simulink model "TVCVehicleModelAndSimulation_AreaVersion"  (R2024a)
settings: Solver=VariableStepAuto  StartTime=0.0  StopTime=20  RelTol=1e-3
values from neighbouring files (symbols this model uses):
  Gravity_Vector_Inertial = [0,0,Mass*9.81]    [ModelVariables.m]
  Thrust_Moment_Arm = 0.1    [ModelVariables.m]
  z_Reference = 30    [ModelVariables.m]
libraries: simulink_extras x2, shared6dof x1, slpidlib x1
settings Model: Creator=Joshua Caratao  LastModifiedBy=Joshua Caratao

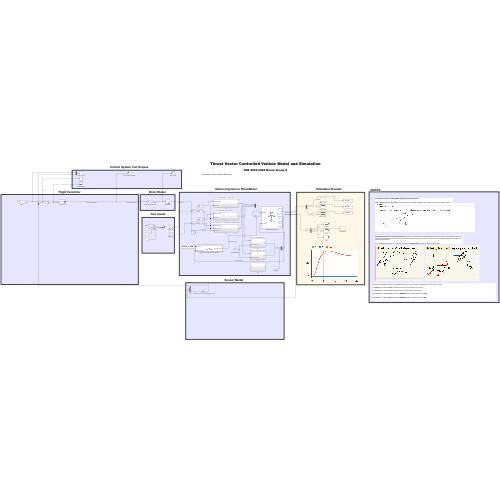
[thumbnail: Simulink's stored preview of the top-level diagram]
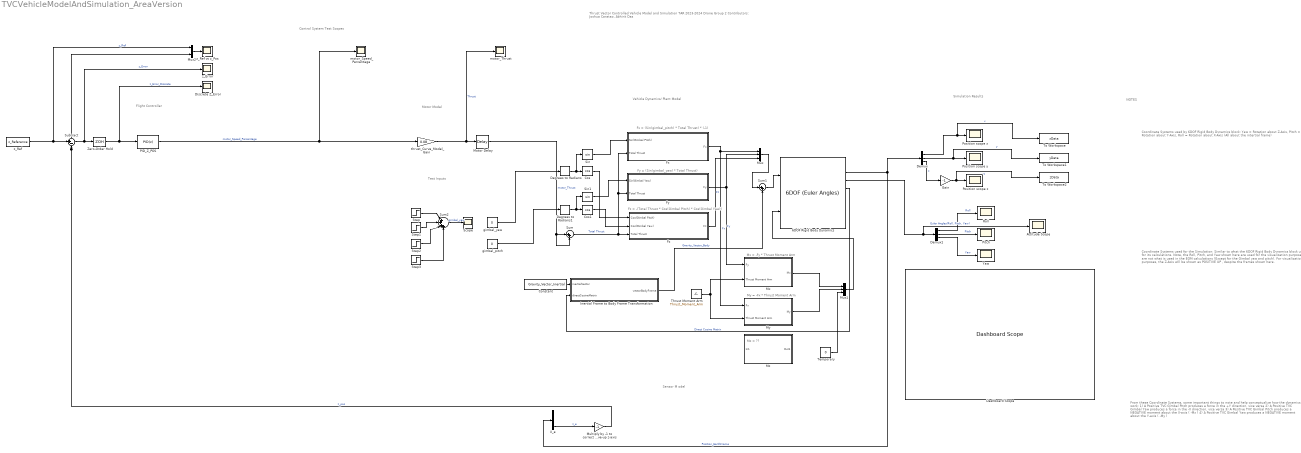
== system TVCVehicleModelAndSimulation_AreaVersion ==
  note: From these Coordinate Systems, some important things to note and help conceptualize how the dynamics work:
      |
      | 1) A Positive TVC Gimbal Pitch produces a force in the +Y direction, vice versa
      |
      | 2) A Positive TVC Gimbal Yaw produces a force in the -X direction, vice versa
      |
      | 3) A Positive TVC Gimbal Pitch produces a NEGATIVE moment about the X-axis ( -Mx )
      |
      | 4) A Positive TVC Gimbal Yaw produces a NEGATIVE moment about the Y-axis ( -My )
  note: NOTES
  note: Coordinate Systems used by 6DOF Rigid Body Dynamics block:
      |
      | Yaw = Rotation about Z-Axis, Pitch = Rotation about Y-Axis, Roll = Rotation about X-Axis (All about the intertial frame)
  note: Coordinate Systems used for the Simulation: Similar to what the 6DOF Rigid Body Dynamics block uses for its calculations. Note, the Roll, Pitch, and Yaw shown here are used for the visualization purposes and are not what is used in the EOM calculations (Except for the Gimbal yaw and pitch).
      |
      | For visualization purposes, the Z-Axis will be shown as POSITIVE UP , despite the frames shown here.
  note: Flight Controller
  note: Sensor M odel
  note: Vehicle Dynamics/ Plant Model
  note: Thrust Vector Controlled Vehicle Model and Simulation
      |
      | TAR 2023-2024 Drone Group 2
      |
      | Contributors: Joshua Caratao, Abhirit Das
  note: Fy = (Sin(gimbal_yaw) * Total Thrust)
  note: My = -Fx * Thrust Moment Arm
  note: Fx = (Sin(gimbal_pitch) * Total Thrust) * (-1)
  note: Mz = ??
  note: Fz = -(Total Thrust * Cos(Gimbal Pitch) * Cos(Gimbal Yaw))
  note: Mx = -Fy * Thrust Moment Arm
  note: Simulation Results
  note: Test Inputs
  note: Motor Model
  note: Control System Test Scopes
  "6DOF Rigid Body Dynamics " : shared6dof/6DOF (Euler Angles)  units=Metric (MKS)  mtype=Fixed  rep=Euler Angles  xme_0=Initial_Pos_Inertial_Axes  Vm_0=Initial_Vel_Body_Axes  eul_0=Initial_Euler_Orientation  pm_0=Initial_Body_Rotation_Rates  mass_0=Mass  mass_e=0.5  mass_f=2.0  inertia=Inertia_Tensor  inertia_e=eye(3)  inertia_f=2*eye(3)  k_quat=1.0  vre_flag=on  abi_flag=off  aMode=0  xme_statename=''  Vm_statename=''  eul_statename=''  quat_statename=''  pm_statename=''  mass_statename=''
  Attitude Scope : Scope
  Constant : Constant  Value=Gravity_Vector_Inertial
  Cos : Trigonometry  Operator=cos
  Cos1 : Trigonometry  Operator=cos
  Dashboard Scope : DashboardScope
  Degrees to Radians : simulink_extras/Transformations/Degrees to Radians
  Degrees to Radians1 : simulink_extras/Transformations/Degrees to Radians
  Demux : Demux  Outputs=3
  Demux1 : Demux  Outputs=3
  Discrete Z_Error : Scope
  Fx : Subsystem
  Fy : Subsystem
  Fz : Subsystem
  Gain : Gain  Gain=-1
  Inertial Frame to Body Frame Transformation : MATLAB Function  TreatAsAtomicUnit=on
  Motor Delay : TransportDelay  DelayTime=0.01
  Multiply by -1 to correct for a positive-up z-axis : Gain  Gain=-1
  Mux : Mux  Inputs=3
  Mux1 : Mux  Inputs=3
  Mux2 : Mux  Inputs=2
  Mx : Subsystem
  My : Subsystem
  Mz : Subsystem
  PID_Z_POS : slpidlib/PID Controller  Controller=PID  Form=Parallel  TimeDomain=Discrete-time  UseExternalTs=off  SampleTime=-1  IntegratorMethod=Forward Euler  FilterMethod=Forward Euler  ControllerParametersSource=internal  P=20  I=4  UseKiTs=off  D=40  UseExternalDerivativeSource=off  N=0  UseFilter=off  TunerSelectOption=Transfer Function Based (PID Tuner App)  InitialConditionSource=internal  InitialConditionForIntegrator=0  InitialConditionForFilter=0  DifferentiatorICPrevScaledInput=0  ExternalReset=none  TrackingMode=off  Kt=1  LimitOutput=on  SatLimitsSource=internal  UpperSaturationLimit=100  LowerSaturationLimit=0  LinearizeAsGain=off  AntiWindupMode=none  Kb=1  LimitIntegrator=off  UpperIntegratorSaturationLimit=2000  LowerIntegratorSaturationLimit=1000  POutMin=[]  POutMax=[]  IOutMin=[]  IOutMax=[]  DOutMin=[]  DOutMax=[]  NOutMin=[]  NOutMax=[]  SumOutMin=[]  SumOutMax=[]  SaturationOutMin=[]  SaturationOutMax=[]  PParamMin=[]  PParamMax=[]  IParamMin=[]  IParamMax=[]  DParamMin=[]  DParamMax=[]  NParamMin=[]  NParamMax=[]  KbParamMin=[]  KbParamMax=[]  KtParamMin=[]  KtParamMax=[]  KbOutMin=[]  KbOutMax=[]  KtOutMin=[]  KtOutMax=[]  IntegratorOutMin=[]  IntegratorOutMax=[]  FilterOutMin=[]  FilterOutMax=[]  SumI1OutMin=[]  SumI1OutMax=[]  SumI2OutMin=[]  SumI2OutMax=[]  SumI3OutMin=[]  SumI3OutMax=[]  SumI4OutMin=[]  SumI4OutMax=[]  SumDOutMin=[]  SumDOutMax=[]  DifferentiatorOutMin=[]  DifferentiatorOutMax=[]  FilterDiffOutCoefMin=[]  FilterDiffOutCoefMax=[]  ReciprocalOutMin=[]  ReciprocalOutMax=[]  SumDenOutMin=[]  SumDenOutMax=[]  SumNumOutMin=[]  SumNumOutMax=[]  DivideOutMin=[]  DivideOutMax=[]  UdiffTsProdOutMin=[]  UdiffTsProdOutMax=[]  NTsProdOutMin=[]  NTsProdOutMax=[]  UintegralTsProdOutMin=[]  UintegralTsProdOutMax=[]  UngainTsProdOutMin=[]  UngainTsProdOutMax=[]  ClampingZeroOutDataTypeStr=Inherit: Inherit via back propagation  ClampingZeroOutMin=[]  ClampingZeroOutMax=[]  FilterDenConstantOutDataTypeStr=Inherit: Inherit via back propagation  FilterDenConstantOutMin=[]  FilterDenConstantOutMax=[]  PCopyOutDataTypeStr=Inherit: Inherit via back propagation  PCopyOutMin=[]  PCopyOutMax=[]  NCopyOutDataTypeStr=Inherit: Inherit via back propagation  NCopyOutMin=[]  NCopyOutMax=[]  IntegratorContinuousStateAttributes=''  IntegratorStateMustResolveToSignalObject=off  IntegratorRTWStateStorageClass=Auto  FilterContinuousStateAttributes=''  FilterStateMustResolveToSignalObject=off  FilterRTWStateStorageClass=Auto  ParallelPVariant=InternalParameters  IdealPVariant=Disabled  IVariant=InternalParameters  DVariant=InternalParameters  IntegratorVariant=Discrete  SatVariant=Enabled  AWVariant=Passthrough  PCopyVariant=Disabled  TRVariant=Disabled  FdbkBlocksVariant=Forward  IdealPFdbkVariant=Disabled  SatFdbkVariant=Disabled  DerivativeFilterVariant=Differentiator  NVariant=Passthrough  NCopyVariant=Disabled_SignalSpec  FilterICVariant=InternalICsDifferentiator  IntegratorICVariant=InternalICs  ExternalResetVariant=Disabled  TRSumVariant=Passthrough  SumFdbkVariant=Disabled  SumVariant=Sum_PID  TsampFilterVariant=InternalTs  TsampNgainVariant=Passthrough  TsampIntegralVariant=Disabled_SignalSpec  ExternalSaturationOutDataTypeStr=Inherit: Same as second input  DerivativeSourceVariant=ErrorSignal
      settings: LibrarySourceBlock=simulink/Discrete/Discrete PID Controller
  Pitch : Scope
  Position scope x : Scope
  Position scope y : Scope
  Position scope z : Scope
  Roll : Scope
  Scope : Scope
  Sin : Trigonometry
  Sin1 : Trigonometry
  Step : Step  SampleTime=0
  Step1 : Step  Time=2  After=-1  SampleTime=0
  Step2 : Step  Time=3  After=-1.5  SampleTime=0
  Step3 : Step  Time=4  After=1.5  SampleTime=0
  Subtract : Sum  Inputs=|+-
  Sum : Sum  Inputs=|++
  Sum1 : Sum  Inputs=|++
  Sum2 : Sum  Inputs=|++++
  Temporary : Constant  Value=0
  "Thrust Moment Arm " : Constant  Value=Thrust_Moment_Arm
  To Workspace : ToWorkspace  VariableName=xData  SampleTime=-1
  To Workspace1 : ToWorkspace  VariableName=yData  SampleTime=-1
  To Workspace2 : ToWorkspace  VariableName=zData  SampleTime=-1
  X_e : Demux  Outputs=3
  Yaw : Scope
  Zero-Order Hold : ZeroOrderHold  SampleTime=0.01
  gimbal_pitch : Constant  Value=0
  gimbal_yaw : Constant  Value=0
  motor_Speed_Percentage : Scope
  motor_Thrust : Scope
  thrust_Curve_Model_Gain : Gain  Gain=0.08
  z_Error : Scope
  z_Ref : Constant  Value=z_Reference
  z_Ref vs z_Pos : Scope
  wires:
  "6DOF Rigid Body Dynamics "/3 -> Attitude Scope/1, Demux1/1  "Euler Angles(Roll, Pitch, Yaw)"
  "6DOF Rigid Body Dynamics "/2 -> X_e/1, Demux/1  "Position_EarthFrame"
  Demux/1 -> To Workspace/1, Position scope x/1  "x"
  Demux/2 -> To Workspace1/1, Position scope y/1  "y"
  Demux/3 -> Gain/1  "z"
  Temporary/1 -> Mux1/3
  "Thrust Moment Arm "/1 -> Mx/2(Thrust Moment Arm), My/2(Thrust Moment Arm)
  My/1(My) -> Mux1/2
  Sin1/1 -> Fy/1(Sin(Gimbal Yaw))
  Fz/1(Fz) -> Mux/3  "Fz"
  Cos1/1 -> Fz/2(Cos(Gimbal Yaw))
  Cos/1 -> Fz/1(Cos(Gimbal Pitch))
  Mx/1(Mx) -> Mux1/1
  Degrees to Radians1/1 -> Sin1/1, Cos1/1
  Sum2/1 -> Scope/1  "gimbal_yaw"
  Mux1/1 -> "6DOF Rigid Body Dynamics "/2
  Fy/1(Fy) -> Mux/2, Mx/1(Fy)  "Fy"
  gimbal_pitch/1 -> Degrees to Radians1/1
  Mux/1 -> Sum1/1
  Sum/1 -> Fz/3(Total Thrust), Fx/2(Total Thrust), Fy/2(Total Thrust)  "Total Thrust"
  Sin/1 -> Fx/1(Sin(Gimbal Pitch))
  Degrees to Radians/1 -> Sin/1, Cos/1
  Fx/1(Fx) -> Mux/1, My/1(Fx)  "Fx"
  thrust_Curve_Model_Gain/1 -> Motor Delay/1, motor_Thrust/1  "Thrust"
  Demux1/2 -> Pitch/1  "Pitch"
  Demux1/1 -> Roll/1  "Roll"
  Demux1/3 -> Yaw/1  "Yaw"
  Sum1/1 -> "6DOF Rigid Body Dynamics "/1
  Inertial Frame to Body Frame Transformation/1(vectorBodyFrame) -> Sum1/2  "Gravity_Vector_Body"
  "6DOF Rigid Body Dynamics "/4 -> Inertial Frame to Body Frame Transformation/2(directCosineMatrix)  "Direct Cosine Matrix"
  Constant/1 -> Inertial Frame to Body Frame Transformation/1(inertialVector)
  Gain/1 -> To Workspace2/1, Position scope z/1  "-z"
  Step/1 -> Sum2/1
  Step1/1 -> Sum2/2
  Step2/1 -> Sum2/3
  Step3/1 -> Sum2/4
  Subtract/1 -> z_Error/1, Zero-Order Hold/1  "z_Error"
  Zero-Order Hold/1 -> Discrete Z_Error/1, PID_Z_POS/1  "z_Error_Discrete"
  PID_Z_POS/1 -> motor_Speed_Percentage/1, thrust_Curve_Model_Gain/1  "motor_Speed_Percentage"
  gimbal_yaw/1 -> Degrees to Radians/1
  Mux2/1 -> z_Ref vs z_Pos/1
  X_e/3 -> Multiply by -1 to correct for a positive-up z-axis/1  "z_e"
  Multiply by -1 to correct for a positive-up z-axis/1 -> Mux2/2, Subtract/2  "z_pos"
  Motor Delay/1 -> Sum/2, Sum/1  "motor_Thrust"
  z_Ref/1 -> Mux2/1, Subtract/1  "z_Ref"

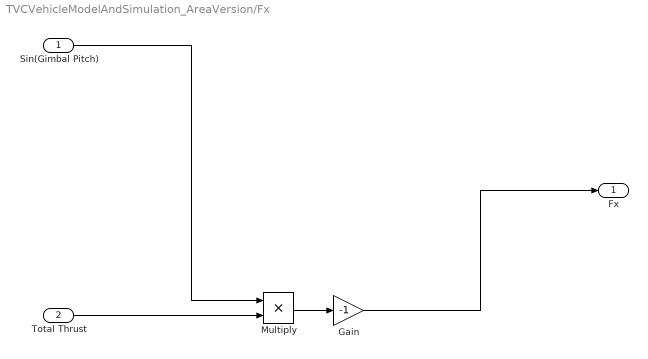
== system TVCVehicleModelAndSimulation_AreaVersion/Fx ==
  Sin(Gimbal Pitch) : Inport
  Total Thrust : Inport  Port=2
  Gain : Gain  Gain=-1
  Multiply : Product
  Fx : Outport
  wires:
  Multiply/1 -> Gain/1
  Sin(Gimbal Pitch)/1 -> Multiply/1
  Total Thrust/1 -> Multiply/2
  Gain/1 -> Fx/1

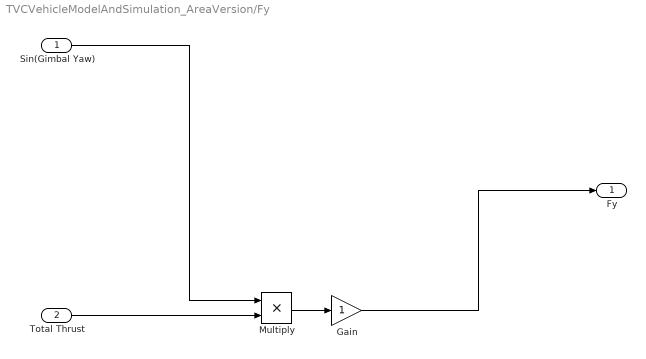
== system TVCVehicleModelAndSimulation_AreaVersion/Fy ==
  Sin(Gimbal Yaw) : Inport
  Total Thrust : Inport  Port=2
  Gain : Gain
  Multiply : Product
  Fy : Outport
  wires:
  Multiply/1 -> Gain/1
  Sin(Gimbal Yaw)/1 -> Multiply/1
  Total Thrust/1 -> Multiply/2
  Gain/1 -> Fy/1

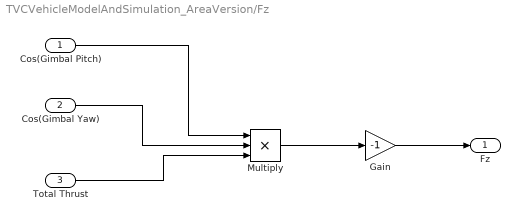
== system TVCVehicleModelAndSimulation_AreaVersion/Fz ==
  Cos(Gimbal Pitch) : Inport
  Cos(Gimbal Yaw) : Inport  Port=2
  Total Thrust : Inport  Port=3
  Gain : Gain  Gain=-1
  Multiply : Product  Inputs=3
  Fz : Outport
  wires:
  Cos(Gimbal Pitch)/1 -> Multiply/1
  Cos(Gimbal Yaw)/1 -> Multiply/2
  Multiply/1 -> Gain/1
  Total Thrust/1 -> Multiply/3
  Gain/1 -> Fz/1

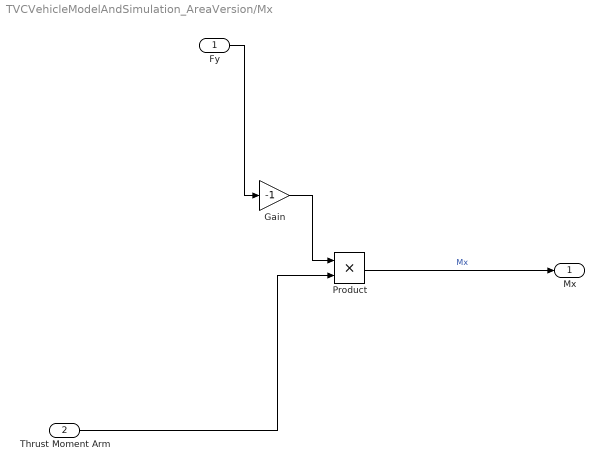
== system TVCVehicleModelAndSimulation_AreaVersion/Mx ==
  Fy : Inport
  Thrust Moment Arm : Inport  Port=2
  Gain : Gain  Gain=-1
  Product : Product
  Mx : Outport
  wires:
  Thrust Moment Arm/1 -> Product/2
  Fy/1 -> Gain/1
  Product/1 -> Mx/1  "Mx"
  Gain/1 -> Product/1

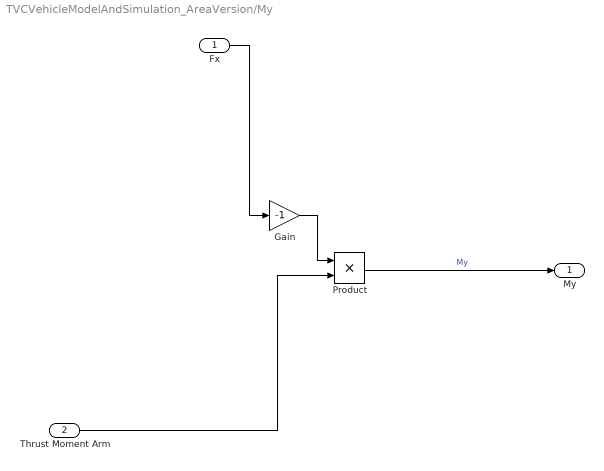
== system TVCVehicleModelAndSimulation_AreaVersion/My ==
  Fx : Inport
  Thrust Moment Arm : Inport  Port=2
  Gain : Gain  Gain=-1
  Product : Product
  My : Outport
  wires:
  Thrust Moment Arm/1 -> Product/2
  Fx/1 -> Gain/1
  Product/1 -> My/1  "My"
  Gain/1 -> Product/1

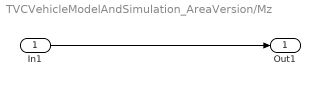
== system TVCVehicleModelAndSimulation_AreaVersion/Mz ==
  In1 : Inport
  Out1 : Outport
  wires:
  In1/1 -> Out1/1

== matlab function TVCVehicleModelAndSimulation_AreaVersion/Inertial Frame to Body Frame Transformation ==
  data: inertialVector input; vectorBodyFrame output; directCosineMatrix input
function vectorBodyFrame = inertialToBodyFrame(inertialVector, directCosineMatrix)
    % Function to transform a vector from the inertial frame to the body-fixed frame
    % using Direct Cosine Matrix.
    %
    % Inputs:
    %   inertial_vector - 3x1 vector in the inertial frame
    %   directCosineMatrix - 3x3 vector that represents orientation and can be used to perform coordinate transformations
    
   
    % Output:
    %   vectorBodyFrame - 3x1 vector in the body-fixed frame


    % % Define the rotation matrices
    % R1_roll = [1, 0, 0;
    %            0, cos(roll), sin(roll);
    %            0, -sin(roll), cos(roll)];
    % 
    % R2_pitch = [cos(pitch), 0, -sin(pitch);
    %             0, 1, 0;
    %             sin(pitch), 0, cos(pitch)];
    % 
    % R3_yaw = [cos(yaw), sin(yaw), 0;
    %           -sin(yaw), cos(yaw), 0;
    %           0, 0, 1];
    % 
    % % Composite rotation matrix
    % R = R1_roll * R2_pitch * R3_yaw;
    


    % Transform the vector using DCM
   vectorBodyFrame = directCosineMatrix * inertialVector;
   
end
